simulink model "PMSM_Simulink_Model"  (Simulink 7.7)
settings: Solver=ode3  StartTime=0.0  StopTime=2  FixedStep=1e-4  RelTol=1e-3
PreLoadFcn:
  | PMSM_Control_Cont_Init
values from neighbouring files (symbols this model uses):
  J = .001    (= 0.001)    [Motor_Parameter.m]
undefined symbols (not defined in the file or in its folder): L_sd, L_sq, p, Psi_R, R_s
settings Model: Creator=schoeatu  LastModifiedBy=Sayed

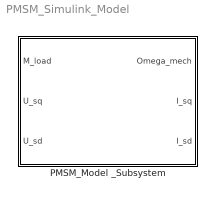
== system PMSM_Simulink_Model ==
  PMSM_Model _Subsystem : Subsystem
      mask Display:
      | port_label('input', 1, 'M_load')
      | port_label('input', 2, 'U_sq')
      | port_label('input', 3, 'U_sd')
      | port_label('output', 1, 'Omega_mech')
      | port_label('output', 2, 'I_sq')
      | port_label('output', 3, 'I_sd')

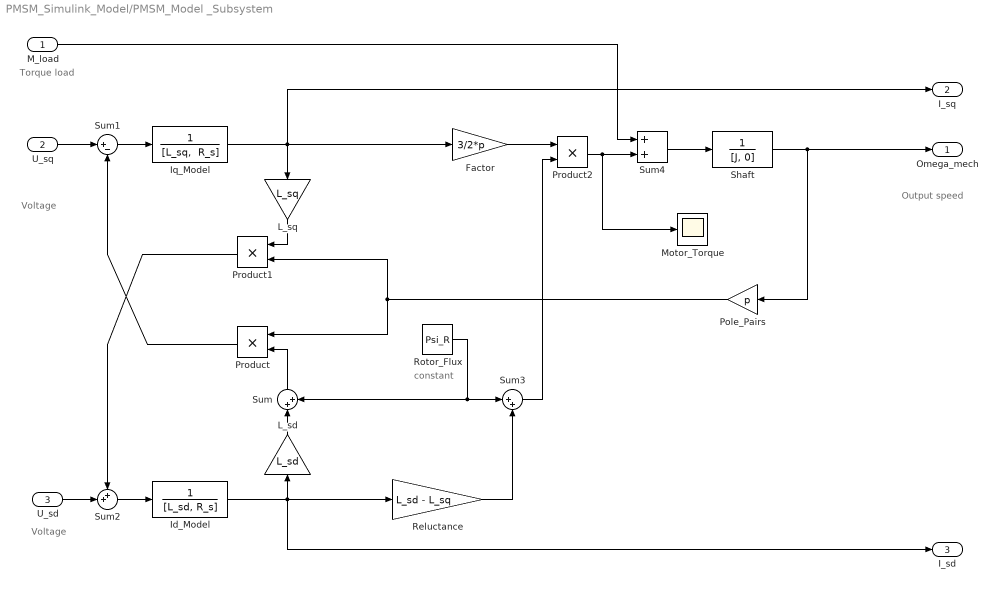
== system PMSM_Simulink_Model/PMSM_Model _Subsystem ==
  note: Voltage
  note: Torque load
  note: Voltage
  note: Output speed
  note: constant
  M_load : Inport
  U_sq : Inport  Port=2
  U_sd : Inport  Port=3
  Factor : Gain  Gain=3/2*p
  Id_Model : TransferFcn  Denominator=[L_sd, R_s]
  Iq_Model : TransferFcn  Denominator="[L_sq,  R_s]"
  L_sd : Gain  Gain=L_sd
  L_sq : Gain  Gain=L_sq
  Motor_Torque : Scope
      settings: TimeRange=2  YMin=-2  YMax=16  SaveName=ScopeData5
  Pole_Pairs : Gain  Gain=p
  Product : Product  RndMeth=Zero
  Product1 : Product  RndMeth=Zero
  Product2 : Product  RndMeth=Zero
  Reluctance : Gain  Gain=L_sd - L_sq
  Rotor_Flux : Constant  Value=Psi_R
  Shaft : TransferFcn  Denominator=[J, 0]
  Sum : Sum  Inputs=|++
  Sum1 : Sum  Inputs=|+-
  Sum2 : Sum  Inputs=++|
  Sum3 : Sum  Inputs=|++
  Sum4 : Sum
  Omega_mech : Outport
  I_sq : Outport  Port=2
  I_sd : Outport  Port=3
  wires:
  Iq_Model/1 -> L_sq/1, Factor/1, I_sq/1
  Id_Model/1 -> L_sd/1, Reluctance/1, I_sd/1
  L_sd/1 -> Sum/1
  Rotor_Flux/1 -> Sum/2, Sum3/1
  Pole_Pairs/1 -> Product/1, Product1/2
  Sum1/1 -> Iq_Model/1
  L_sq/1 -> Product1/1
  Sum2/1 -> Id_Model/1
  Product1/1 -> Sum2/1
  Reluctance/1 -> Sum3/2
  M_load/1 -> Sum4/1
  Sum4/1 -> Shaft/1
  Shaft/1 -> Pole_Pairs/1, Omega_mech/1
  U_sq/1 -> Sum1/1
  U_sd/1 -> Sum2/2
  Product2/1 -> Sum4/2, Motor_Torque/1
  Factor/1 -> Product2/1
  Sum3/1 -> Product2/2
  Sum/1 -> Product/2
  Product/1 -> Sum1/2
